simulink model "momentum_dump_test_rev2"  (R2016b)
settings: Solver=VariableStepAuto  StartTime=0.0  StopTime=5400  MinStep=0.001  RelTol=1e-3
values from neighbouring files (symbols this model uses):
  fsw_params = init_fsw_params()    [momentum_unload_test_init.m]
libraries: dynamics_lib x1, environment_lib x1, momentum_dump_lib x1, pd_control_lib x1, aerolibutil x1, RW_assembly_simple_lib x1, command_processing x1, magnetorquer_assembly_lib x1
settings Model: Creator=evich  LastModifiedBy=Taylor

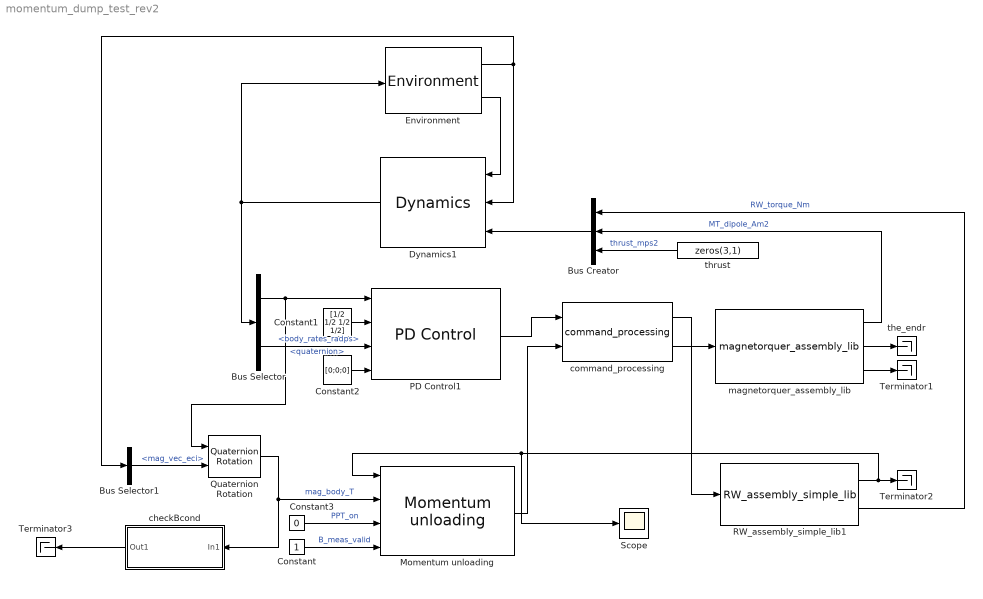
== system momentum_dump_test_rev2 ==
  Bus Creator : BusCreator  Inputs=3
  Bus Selector : BusSelector  OutputSignals=quaternion,body_rates_radps
  Bus Selector1 : BusSelector  OutputSignals=mag_vec_eci
  Constant : Constant
  Constant1 : Constant  Value=[1/2 1/2 1/2 1/2]
  Constant2 : Constant  Value=[0;0;0]
  Constant3 : Constant  Value=0
  Dynamics1 : dynamics_lib/Dynamics
  Environment : environment_lib/Environment
  Momentum unloading : momentum_dump_lib/Momentum unloading
  PD Control1 : pd_control_lib/PD Control
  Quaternion Rotation : aerolibutil/Quaternion Rotation
  RW_assembly_simple_lib1 : RW_assembly_simple_lib/RW_assembly_simple_lib  natural_frequency=sim_params.actuators.reaction_wheel.natural_freq  damping_ratio=sim_params.actuators.reaction_wheel.damping  max_rate=sim_params.actuators.reaction_wheel.rate_limit
  Scope : Scope
  Terminator1 : Terminator
  Terminator2 : Terminator
  Terminator3 : Terminator
  checkBcond : Subsystem
  command_processing : command_processing/command_processing
  magnetorquer_assembly_lib : magnetorquer_assembly_lib/magnetorquer_assembly_lib
  the_endr : Terminator
  thrust : Constant  Value=zeros(3,1)
  wires:
  Dynamics1/1 -> Environment/1, Bus Selector/1
  Environment/2 -> Dynamics1/1
  Environment/1 -> Bus Selector1/1, Dynamics1/2
  Bus Creator/1 -> Dynamics1/3
  RW_assembly_simple_lib1/2 -> Bus Creator/1  "RW_torque_Nm"
  magnetorquer_assembly_lib/1 -> Bus Creator/2  "MT_dipole_Am2"
  Bus Selector/1 -> PD Control1/1, Quaternion Rotation/1  "<quaternion>"
  Bus Selector/2 -> PD Control1/3  "<body_rates_radps>"
  command_processing/1 -> RW_assembly_simple_lib1/1
  command_processing/2 -> magnetorquer_assembly_lib/1
  Constant3/1 -> Momentum unloading/3  "PPT_on"
  Constant/1 -> Momentum unloading/4  "B_meas_valid"
  Constant1/1 -> PD Control1/2
  Constant2/1 -> PD Control1/4
  magnetorquer_assembly_lib/2 -> the_endr/1
  magnetorquer_assembly_lib/3 -> Terminator1/1
  RW_assembly_simple_lib1/1 -> Scope/1, Momentum unloading/1, Terminator2/1
  Bus Selector1/1 -> Quaternion Rotation/2  "<mag_vec_eci>"
  Quaternion Rotation/1 -> Momentum unloading/2, checkBcond/1(In1)  "mag_body_T"
  Momentum unloading/1 -> command_processing/2
  PD Control1/1 -> command_processing/1
  checkBcond/1(Out1) -> Terminator3/1
  thrust/1 -> Bus Creator/3  "thrust_mps2"

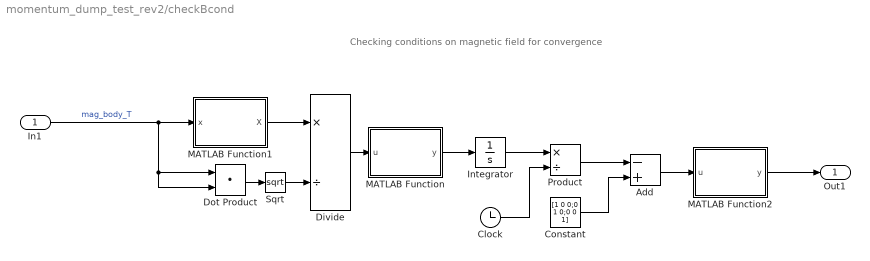
== system momentum_dump_test_rev2/checkBcond ==
  note: Checking conditions on magnetic field for convergence
  In1 : Inport
  Add : Sum  Inputs=-+
  Clock : Clock
      settings: Decimation=10000
  Constant : Constant  Value=[1 0 0;0 1 0;0 0 1]
  Divide : Product  Inputs=*/
  Dot Product : DotProduct  InputSameDT=on  OutDataTypeStr=Inherit: Inherit via internal rule
  Integrator : Integrator  InitialCondition=fsw_params.control.p_dump.ic.delay_B*fsw_params.control.p_dump.ic.delay_B'
  MATLAB Function : MATLAB Function  TreatAsAtomicUnit=on
  MATLAB Function1 : MATLAB Function  TreatAsAtomicUnit=on
  MATLAB Function2 : MATLAB Function  TreatAsAtomicUnit=on
  Product : Product  Inputs=*/
  Sqrt : Sqrt  SaturateOnIntegerOverflow=on
  Out1 : Outport
  wires:
  In1/1 -> Dot Product/2, Dot Product/1, MATLAB Function1/1(x)  "mag_body_T"
  MATLAB Function/1(y) -> Integrator/1
  Integrator/1 -> Product/1
  Clock/1 -> Product/2
  Dot Product/1 -> Sqrt/1
  MATLAB Function1/1(X) -> Divide/1
  Divide/1 -> MATLAB Function/1(u)
  Sqrt/1 -> Divide/2
  Product/1 -> Add/1
  Constant/1 -> Add/2
  Add/1 -> MATLAB Function2/1(u)
  MATLAB Function2/1(y) -> Out1/1

== matlab function momentum_dump_test_rev2/checkBcond/MATLAB Function ==
  data: u input; y output
function y = outerprod(u)

y = u*u';

== matlab function momentum_dump_test_rev2/checkBcond/MATLAB Function1 ==
  data: x input; X output
function X   = skew( x )
% UW HuskySat-1, ADCS Subsystem
% Last Update: E. Hansen 12.8.2017

%Transforms a vector into a skew symmetric matrix (Levi-Civita)
%--------------------------------------------------------------------------

X = [0 -x(3) x(2);x(3) 0 -x(1);-x(2) x(1) 0];

== matlab function momentum_dump_test_rev2/checkBcond/MATLAB Function2 ==
  data: u input; y output
function y = eigval(u)

y = eig(u);
